simulink model "chapter2_4_1"  (R2022a)
settings: Solver=FixedStepAuto  StartTime=0.0  StopTime=8  FixedStep=1e-3  RelTol=1e-3
model workspace (MAT data in the model file):
  maxRandom = 1e-06
  minRandom = -1e-06
values from neighbouring files (symbols this model uses):
  Cb = 11e3    (= 11000)    [parameterLoadForchapter2_4.m]    (also in parameterLoadForchapter2_5.m)
  Cv = 5000    [parameterLoadForchapter2_4.m]    (also in parameterLoadForchapter2_5.m)
  d = 2.6    [parameterLoadForchapter2_4.m]    (also in parameterLoadForchapter2_5.m; parameter_load3.m)
  Jb = 927.8    [parameterLoadForchapter2_4.m]    (also in parameterLoadForchapter2_5.m)
  Jv = 3044    [parameterLoadForchapter2_4.m]    (also in parameterLoadForchapter2_5.m)
  Kb = 0.267e6    (= 267000)    [parameterLoadForchapter2_4.m]    (also in parameterLoadForchapter2_5.m)
  Kv = 1.5e6    (= 1500000)    [parameterLoadForchapter2_4.m]    (also in parameterLoadForchapter2_5.m)
  L = 210/2    (= 105)    [Figure2_18_and2_19.m]    (also in Figure2_20_and2_21.m; parameterLoadForchapter2_4.m = 15.6; parameterLoadForchapter2_5.m = 210; parameter_load3.m = 210)
  Ln = Lns(i)    [Figure2_14and2_15.m]    (also in Figure2_16and2_17.m; Mchapter2_4.m = LNs(i); Mchapter2_5.m = LN_set(i); parameterLoadForchapter2_5.m = 0.02)
  Ln1 = Ln    [Figure2_14and2_15.m]    (also in Figure2_16and2_17.m)
  Mb = 23000    [parameterLoadForchapter2_4.m]    (also in parameterLoadForchapter2_5.m)
  Mv = 4060    [parameterLoadForchapter2_4.m]    (also in parameterLoadForchapter2_5.m)
  mw = 1670    [parameterLoadForchapter2_4.m]    (also in parameterLoadForchapter2_5.m)
  Mw = 1670    [parameterLoadForchapter2_4.m]    (also in parameterLoadForchapter2_5.m)
  R = 400    [Figure2_3.m]    (also in parameterLoadForchapter2_4.m = 0.42; parameterLoadForchapter2_5.m = 0.42)
  r = 0.42    [parameterLoadForchapter2_4.m]    (also in parameterLoadForchapter2_5.m; parameter_load3.m)
  vkmh = 50    [parameterLoadForchapter2_4.m]    (also in parameterLoadForchapter2_5.m = 100)
settings Model: Creator=Spicydel  LastModifiedBy=Spicydel

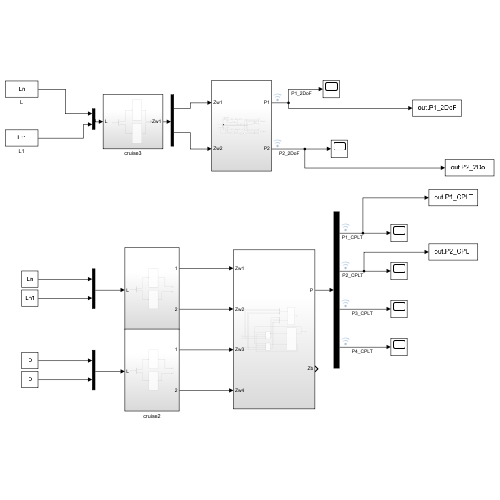
[thumbnail: Simulink's stored preview of the top-level diagram]
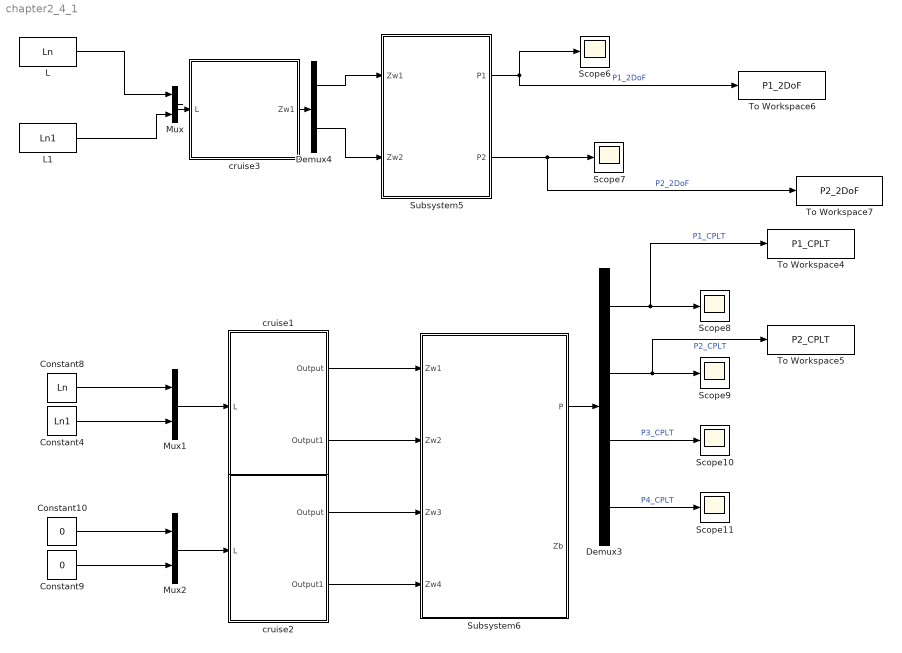
== system chapter2_4_1 ==
  Constant10 : Constant  Value=0
  Constant4 : Constant  Value=Ln1
  Constant8 : Constant  Value=Ln
  Constant9 : Constant  Value=0
  Demux3 : Demux
  Demux4 : Demux  Outputs=2
  L : Constant  Value=Ln
  L1 : Constant  Value=Ln1
  Mux : Mux  Inputs=2
  Mux1 : Mux  Inputs=2
  Mux2 : Mux  Inputs=2
  Scope{6..11} (6 alike) : Scope
  Subsystem5 : Subsystem
  Subsystem6 : Subsystem
  To Workspace4 : ToWorkspace  VariableName=P1_CPLT  SaveFormat=Timeseries  SampleTime=-1
  To Workspace5 : ToWorkspace  VariableName=P2_CPLT  SaveFormat=Timeseries  SampleTime=-1
  To Workspace6 : ToWorkspace  VariableName=P1_2DoF  SaveFormat=Timeseries  SampleTime=-1
  To Workspace7 : ToWorkspace  VariableName=P2_2DoF  SaveFormat=Timeseries  SampleTime=-1
  cruise1 : Subsystem
  cruise2 : Subsystem
  cruise3 : Subsystem
  wires:
  L/1 -> Mux/1
  Subsystem5/2(P2) -> To Workspace7/1, Scope7/1  "P2_2DoF"
  Subsystem5/1(P1) -> To Workspace6/1, Scope6/1  "P1_2DoF"
  Mux/1 -> cruise3/1(L)
  L1/1 -> Mux/2
  Demux4/1 -> Subsystem5/1(Zw1)
  Demux4/2 -> Subsystem5/2(Zw2)
  cruise1/1(Output) -> Subsystem6/1(Zw1)
  cruise1/2(Output1) -> Subsystem6/2(Zw2)
  cruise2/1(Output) -> Subsystem6/3(Zw3)
  cruise2/2(Output1) -> Subsystem6/4(Zw4)
  Constant4/1 -> Mux1/2
  Mux1/1 -> cruise1/1(L)
  Constant8/1 -> Mux1/1
  Constant10/1 -> Mux2/1
  Mux2/1 -> cruise2/1(L)
  Constant9/1 -> Mux2/2
  Demux3/4 -> Scope11/1  "P4_CPLT"
  Demux3/3 -> Scope10/1  "P3_CPLT"
  Demux3/2 -> To Workspace5/1, Scope9/1  "P2_CPLT"
  Demux3/1 -> To Workspace4/1, Scope8/1  "P1_CPLT"
  Subsystem6/1(P) -> Demux3/1
  cruise3/1(Zw1) -> Demux4/1

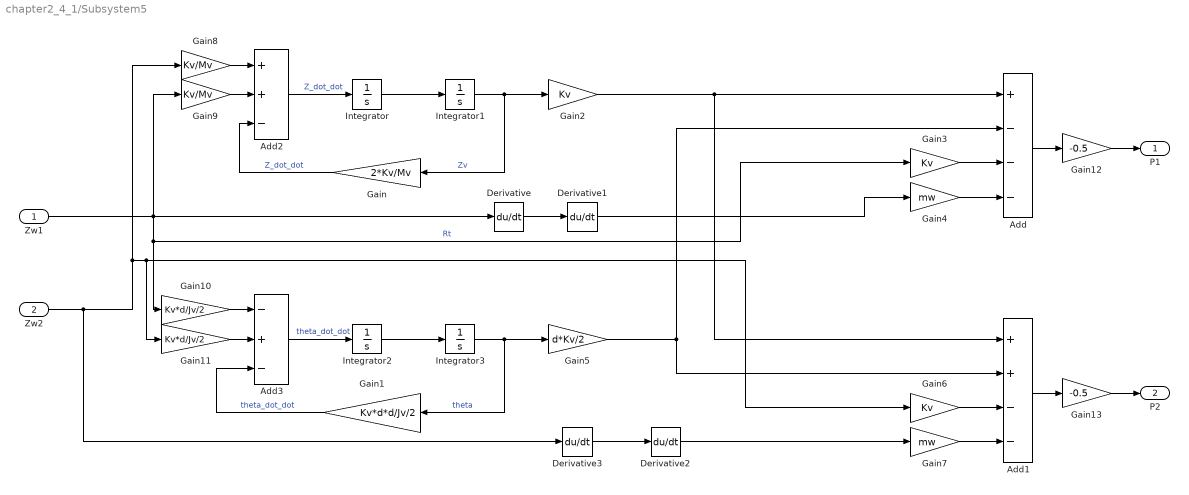
== system chapter2_4_1/Subsystem5 ==
  Zw1 : Inport
  Zw2 : Inport  Port=2
  Add : Sum  Inputs=+---
  Add1 : Sum  Inputs=++--
  Add2 : Sum  Inputs=++-
  Add3 : Sum  Inputs=-+-
  Derivative{,1..3} (4 alike) : Derivative
  Gain : Gain  Gain=2*Kv/Mv
  Gain1 : Gain  Gain=Kv*d*d/Jv/2
  Gain10 : Gain  Gain=Kv*d/Jv/2
  Gain11 : Gain  Gain=Kv*d/Jv/2
  Gain12 : Gain  Gain=-0.5
  Gain13 : Gain  Gain=-0.5
  Gain2 : Gain  Gain=Kv
  Gain3 : Gain  Gain=Kv
  Gain4 : Gain  Gain=mw
  Gain5 : Gain  Gain=d*Kv/2
  Gain6 : Gain  Gain=Kv
  Gain7 : Gain  Gain=mw
  Gain8 : Gain  Gain=Kv/Mv
  Gain9 : Gain  Gain=Kv/Mv
  Integrator{,1..3} (4 alike) : Integrator
  P1 : Outport
  P2 : Outport  Port=2
  wires:
  Gain13/1 -> P2/1
  Gain12/1 -> P1/1
  Gain11/1 -> Add3/2
  Gain10/1 -> Add3/1
  Gain1/1 -> Add3/3  "theta_dot_dot"
  Gain9/1 -> Add2/2
  Gain8/1 -> Add2/1
  Gain/1 -> Add2/3  "Z_dot_dot"
  Gain7/1 -> Add1/4
  Zw2/1 -> Derivative3/1, Gain8/1, Gain6/1, Gain11/1
  Gain6/1 -> Add1/3
  Gain4/1 -> Add/4
  Gain3/1 -> Add/3
  Zw1/1 -> Derivative/1, Gain3/1, Gain10/1, Gain9/1  "Rt"
  Add1/1 -> Gain13/1
  Add/1 -> Gain12/1
  Gain5/1 -> Add1/2, Add/2
  Gain2/1 -> Add/1, Add1/1
  Add3/1 -> Integrator2/1  "theta_dot_dot"
  Integrator3/1 -> Gain1/1, Gain5/1  "theta"
  Integrator2/1 -> Integrator3/1
  Add2/1 -> Integrator/1  "Z_dot_dot"
  Integrator1/1 -> Gain/1, Gain2/1  "Zv"
  Integrator/1 -> Integrator1/1
  Derivative/1 -> Derivative1/1
  Derivative1/1 -> Gain4/1
  Derivative2/1 -> Gain7/1
  Derivative3/1 -> Derivative2/1

== system chapter2_4_1/Subsystem6 ==
  Zw1 : Inport
  Zw2 : Inport  Port=2
  Zw3 : Inport  Port=3
  Zw4 : Inport  Port=4
  FrontTrans : Subsystem
  Mux : Mux
  Mux1 : Mux
  RearTrans : Subsystem
  Subsystem : Subsystem
  Subsystem2 : Subsystem
  P : Outport
  Zb : Outport  Port=2
  wires:
  Subsystem/1(P) -> P/1
  Mux1/1 -> Subsystem/2(Z&theta)
  Mux/1 -> Subsystem/1(Zw)
  RearTrans/2(theta_v2) -> Mux1/4
  FrontTrans/2(theta_v1) -> Mux1/2
  Zw2/1 -> FrontTrans/4(Zw2), Mux/2
  Zw1/1 -> FrontTrans/3(Zw1), Mux/1
  Zw3/1 -> RearTrans/3(Zw3), Mux/3
  Subsystem2/2(theta_b) -> RearTrans/2(theta_b), FrontTrans/2(theta_b)
  Zw4/1 -> RearTrans/4(Zw4), Mux/4
  Subsystem2/1(Zb) -> FrontTrans/1(Zb), RearTrans/1(Zb), Zb/1  "Zb"
  FrontTrans/1(Zv1) -> Subsystem2/1(Zv1), Mux1/1
  RearTrans/1(Zv2) -> Subsystem2/2(Zv2), Mux1/3

== system chapter2_4_1/cruise1 ==
  L : Inport
  Demux : Demux  Outputs=2
  Subsystem1 : Subsystem
  Subsystem2 : Subsystem
  Output : Outport
  Output1 : Outport  Port=2
  wires:
  Subsystem2/1(Output) -> Output1/1
  Subsystem1/1(Output) -> Output/1
  Demux/2 -> Subsystem2/1(In1)
  Demux/1 -> Subsystem1/1(In1)
  L/1 -> Demux/1

== system chapter2_4_1/cruise2 ==
  L : Inport
  Demux : Demux  Outputs=2
  Subsystem1 : Subsystem
  Subsystem2 : Subsystem
  Output : Outport
  Output1 : Outport  Port=2
  wires:
  L/1 -> Demux/1
  Demux/1 -> Subsystem1/1(In1)
  Demux/2 -> Subsystem2/1(In1)
  Subsystem1/1(Output) -> Output/1
  Subsystem2/1(Output) -> Output1/1

== system chapter2_4_1/cruise3 ==
  L : Inport
  Demux : Demux  Outputs=2
  Mux : Mux  Inputs=2
  Subsystem1 : Subsystem
  Subsystem2 : Subsystem
  Zw1 : Outport
  wires:
  L/1 -> Demux/1
  Demux/1 -> Subsystem1/1(In1)
  Demux/2 -> Subsystem2/1(In1)
  Subsystem1/1(Output) -> Mux/1
  Subsystem2/1(Output) -> Mux/2
  Mux/1 -> Zw1/1

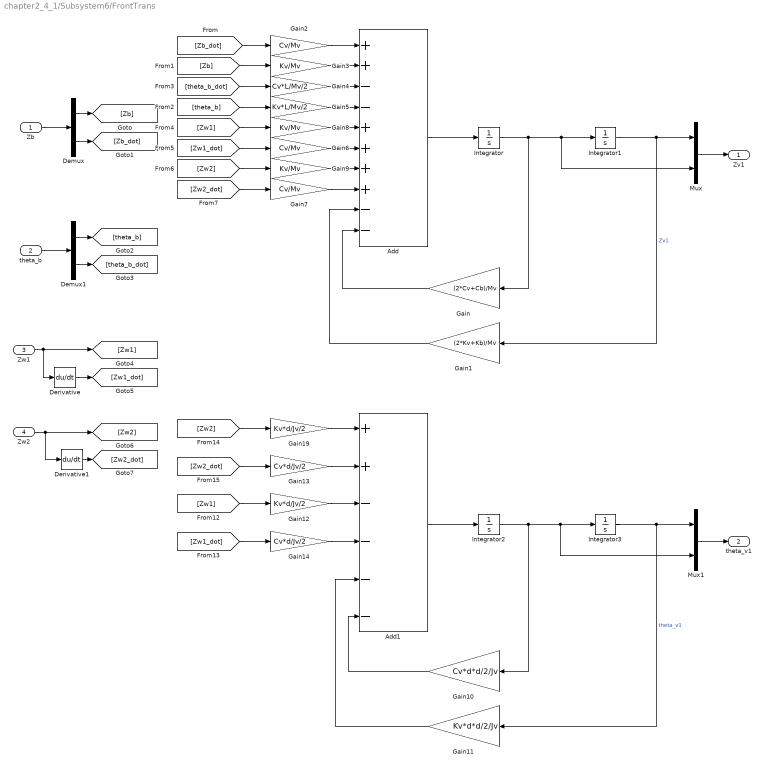
== system chapter2_4_1/Subsystem6/FrontTrans ==
  Zb : Inport
  theta_b : Inport  Port=2
  Zw1 : Inport  Port=3
  Zw2 : Inport  Port=4
  Add : Sum  Inputs=++--++++--
  Add1 : Sum  Inputs=++----
  Demux : Demux  Outputs=2
  Demux1 : Demux  Outputs=2
  Derivative : Derivative
  Derivative1 : Derivative
  Gain : Gain  Gain=(2*Cv+Cb)/Mv
  Gain1 : Gain  Gain=(2*Kv+Kb)/Mv
  Gain10 : Gain  Gain=Cv*d*d/2/Jv
  Gain11 : Gain  Gain=Kv*d*d/2/Jv
  Gain12 : Gain  Gain=Kv*d/Jv/2
  Gain13 : Gain  Gain=Cv*d/Jv/2
  Gain14 : Gain  Gain=Cv*d/Jv/2
  Gain19 : Gain  Gain=Kv*d/Jv/2
  Gain2 : Gain  Gain=Cv/Mv
  Gain3 : Gain  Gain=Kv/Mv
  Gain4 : Gain  Gain=Cv*L/Mv/2
  Gain5 : Gain  Gain=Kv*L/Mv/2
  Gain6 : Gain  Gain=Cv/Mv
  Gain7 : Gain  Gain=Cv/Mv
  Gain8 : Gain  Gain=Kv/Mv
  Gain9 : Gain  Gain=Kv/Mv
  Integrator{,1..3} (4 alike) : Integrator
  Mux : Mux  Inputs=2
  Mux1 : Mux  Inputs=2
  Zv1 : Outport
  theta_v1 : Outport  Port=2
  wires:
  Derivative1/1 -> [Zw2_dot]
  Zw2/1 -> Derivative1/1, [Zw2]
  Derivative/1 -> [Zw1_dot]
  Integrator2/1 -> Gain10/1, Integrator3/1, Mux1/2
  Integrator3/1 -> Gain11/1, Mux1/1  "theta_v1"
  Mux1/1 -> theta_v1/1
  Gain14/1 -> Add1/4
  Gain13/1 -> Add1/2
  Gain12/1 -> Add1/3
  Gain19/1 -> Add1/1
  Add1/1 -> Integrator2/1
  Gain10/1 -> Add1/6
  Gain11/1 -> Add1/5
  [Zw2] -> Gain19/1
  [Zw2_dot] -> Gain13/1
  [Zw1_dot] -> Gain14/1
  [Zw1] -> Gain12/1
  Gain7/1 -> Add/8
  Gain9/1 -> Add/7
  Gain6/1 -> Add/6
  Gain8/1 -> Add/5
  [Zw1] -> Gain8/1
  [Zw1_dot] -> Gain6/1
  [Zw2_dot] -> Gain7/1
  [Zw2] -> Gain9/1
  Gain5/1 -> Add/4
  [theta_b] -> Gain5/1
  Gain4/1 -> Add/3
  [theta_b_dot] -> Gain4/1
  Gain3/1 -> Add/2
  [Zb] -> Gain3/1
  Gain2/1 -> Add/1
  [Zb_dot] -> Gain2/1
  Gain1/1 -> Add/9
  Gain/1 -> Add/10
  Zw1/1 -> Derivative/1, [Zw1]
  Mux/1 -> Zv1/1
  Integrator1/1 -> Mux/1, Gain1/1  "Zv1"
  Add/1 -> Integrator/1
  Integrator/1 -> Integrator1/1, Mux/2, Gain/1
  Demux1/2 -> [theta_b_dot]
  Demux1/1 -> [theta_b]
  Demux/2 -> [Zb_dot]
  Demux/1 -> [Zb]
  theta_b/1 -> Demux1/1
  Zb/1 -> Demux/1

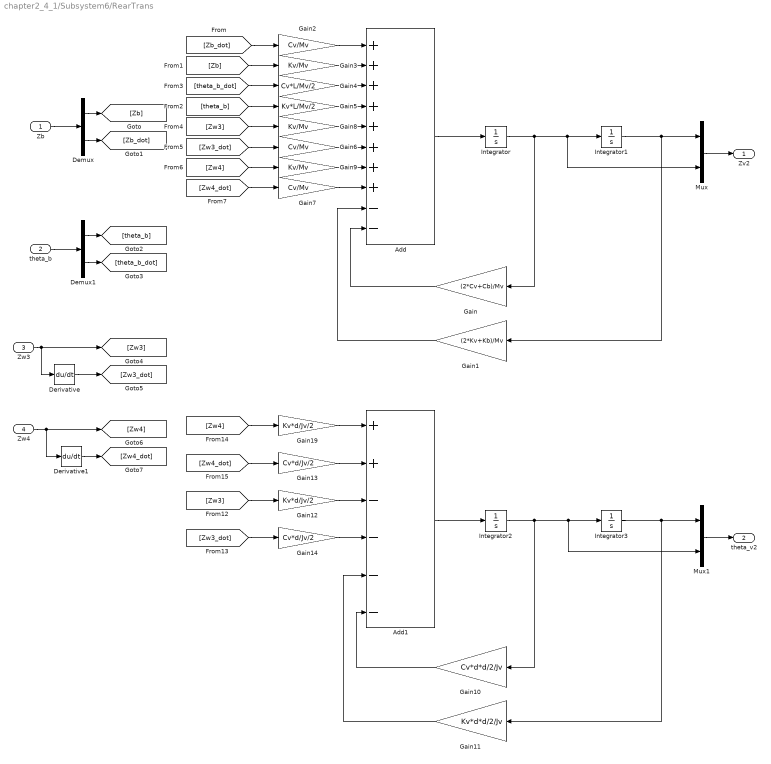
== system chapter2_4_1/Subsystem6/RearTrans ==
  Zb : Inport
  theta_b : Inport  Port=2
  Zw3 : Inport  Port=3
  Zw4 : Inport  Port=4
  Add : Sum  Inputs=++++++++--
  Add1 : Sum  Inputs=++----
  Demux : Demux  Outputs=2
  Demux1 : Demux  Outputs=2
  Derivative : Derivative
  Derivative1 : Derivative
  Gain : Gain  Gain=(2*Cv+Cb)/Mv
  Gain1 : Gain  Gain=(2*Kv+Kb)/Mv
  Gain10 : Gain  Gain=Cv*d*d/2/Jv
  Gain11 : Gain  Gain=Kv*d*d/2/Jv
  Gain12 : Gain  Gain=Kv*d/Jv/2
  Gain13 : Gain  Gain=Cv*d/Jv/2
  Gain14 : Gain  Gain=Cv*d/Jv/2
  Gain19 : Gain  Gain=Kv*d/Jv/2
  Gain2 : Gain  Gain=Cv/Mv
  Gain3 : Gain  Gain=Kv/Mv
  Gain4 : Gain  Gain=Cv*L/Mv/2
  Gain5 : Gain  Gain=Kv*L/Mv/2
  Gain6 : Gain  Gain=Cv/Mv
  Gain7 : Gain  Gain=Cv/Mv
  Gain8 : Gain  Gain=Kv/Mv
  Gain9 : Gain  Gain=Kv/Mv
  Integrator{,1..3} (4 alike) : Integrator
  Mux : Mux  Inputs=2
  Mux1 : Mux  Inputs=2
  Zv2 : Outport
  theta_v2 : Outport  Port=2
  wires:
  Derivative/1 -> [Zw3_dot]
  Mux1/1 -> theta_v2/1
  Integrator3/1 -> Gain11/1, Mux1/1
  Integrator2/1 -> Integrator3/1, Mux1/2, Gain10/1
  Zb/1 -> Demux/1
  theta_b/1 -> Demux1/1
  Demux/1 -> [Zb]
  Demux/2 -> [Zb_dot]
  Demux1/1 -> [theta_b]
  Demux1/2 -> [theta_b_dot]
  Integrator/1 -> Gain/1, Mux/2, Integrator1/1
  Add/1 -> Integrator/1
  Integrator1/1 -> Gain1/1, Mux/1
  Mux/1 -> Zv2/1
  Zw3/1 -> [Zw3], Derivative/1
  Derivative1/1 -> [Zw4_dot]
  Zw4/1 -> [Zw4], Derivative1/1
  Gain/1 -> Add/10
  Gain1/1 -> Add/9
  [Zb_dot] -> Gain2/1
  Gain2/1 -> Add/1
  [Zb] -> Gain3/1
  Gain3/1 -> Add/2
  [theta_b_dot] -> Gain4/1
  Gain4/1 -> Add/3
  [theta_b] -> Gain5/1
  Gain5/1 -> Add/4
  [Zw4] -> Gain9/1
  [Zw4_dot] -> Gain7/1
  [Zw3_dot] -> Gain6/1
  [Zw3] -> Gain8/1
  Gain8/1 -> Add/5
  Gain6/1 -> Add/6
  Gain9/1 -> Add/7
  Gain7/1 -> Add/8
  [Zw3] -> Gain12/1
  [Zw3_dot] -> Gain14/1
  [Zw4_dot] -> Gain13/1
  [Zw4] -> Gain19/1
  Gain11/1 -> Add1/5
  Gain10/1 -> Add1/6
  Add1/1 -> Integrator2/1
  Gain19/1 -> Add1/1
  Gain12/1 -> Add1/3
  Gain13/1 -> Add1/2
  Gain14/1 -> Add1/4

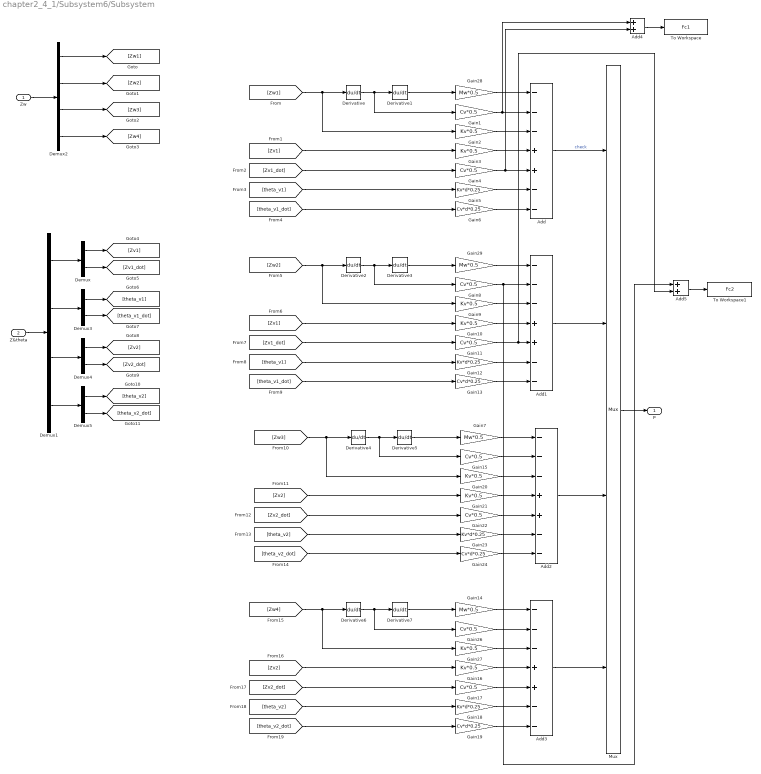
== system chapter2_4_1/Subsystem6/Subsystem ==
  Zw : Inport
  Z&theta : Inport  Port=2
  Add{,1..3} (4 alike) : Sum  Inputs=---++--
  Add4 : Sum
  Add5 : Sum
  Demux{,3..5} (4 alike) : Demux  Outputs=2
  Demux1 : Demux
  Demux2 : Demux
  Derivative{,1..7} (8 alike) : Derivative
  Gain{1,4,8,11,15,17,22,26} (8 alike) : Gain  Gain=Cv*0.5
  Gain{2..3,9..10,16,20..21,27} (8 alike) : Gain  Gain=Kv*0.5
  Gain{5,12,18,23} (4 alike) : Gain  Gain=Kv*d*0.25
  Gain{6,13,19,24} (4 alike) : Gain  Gain=Cv*d*0.25
  Gain{7,14,28..29} (4 alike) : Gain  Gain=Mw*0.5
  Mux : Mux
  To Workspace : ToWorkspace  VariableName=Fc1  SaveFormat=Timeseries  SampleTime=-1
  To Workspace1 : ToWorkspace  VariableName=Fc2  SaveFormat=Timeseries  SampleTime=-1
  P : Outport
  wires:
  Add5/1 -> To Workspace1/1
  Add4/1 -> To Workspace/1
  Mux/1 -> P/1
  [Zw3] -> Derivative4/1, Gain20/1
  Derivative4/1 -> Gain15/1, Derivative5/1
  Derivative5/1 -> Gain7/1
  Gain7/1 -> Add2/1
  Gain15/1 -> Add2/2
  Gain20/1 -> Add2/3
  Gain21/1 -> Add2/4
  [Zv2] -> Gain21/1
  Gain22/1 -> Add2/5
  [Zv2_dot] -> Gain22/1
  Gain23/1 -> Add2/6
  Gain24/1 -> Add2/7
  [theta_v2] -> Gain23/1
  [theta_v2_dot] -> Gain24/1
  Add2/1 -> Mux/3
  Add3/1 -> Mux/4
  [theta_v2_dot] -> Gain19/1
  [theta_v2] -> Gain18/1
  Gain19/1 -> Add3/7
  Gain18/1 -> Add3/6
  [Zv2_dot] -> Gain17/1
  Gain17/1 -> Add3/5
  [Zv2] -> Gain16/1
  Gain16/1 -> Add3/4
  Gain27/1 -> Add3/3
  Gain26/1 -> Add3/2
  Gain14/1 -> Add3/1
  Derivative7/1 -> Gain14/1
  Derivative6/1 -> Derivative7/1, Gain26/1
  [Zw4] -> Derivative6/1, Gain27/1
  [Zw2] -> Derivative2/1, Gain9/1
  Derivative2/1 -> Gain8/1, Derivative3/1
  Derivative3/1 -> Gain29/1
  Gain29/1 -> Add1/1
  Gain8/1 -> Add1/2, Add5/1
  Gain9/1 -> Add1/3
  Gain10/1 -> Add1/4
  [Zv1] -> Gain10/1
  Gain11/1 -> Add1/5, Add5/2
  [Zv1_dot] -> Gain11/1
  Gain12/1 -> Add1/6
  Gain13/1 -> Add1/7
  [theta_v1] -> Gain12/1
  [theta_v1_dot] -> Gain13/1
  Add1/1 -> Mux/2
  Add/1 -> Mux/1  "check"
  [theta_v1_dot] -> Gain6/1
  [theta_v1] -> Gain5/1
  Gain6/1 -> Add/7
  Gain5/1 -> Add/6
  [Zv1_dot] -> Gain4/1
  Gain4/1 -> Add/5, Add4/2
  [Zv1] -> Gain3/1
  Gain3/1 -> Add/4
  Gain2/1 -> Add/3
  Gain1/1 -> Add/2, Add4/1
  Gain28/1 -> Add/1
  Derivative1/1 -> Gain28/1
  Derivative/1 -> Derivative1/1, Gain1/1
  [Zw1] -> Derivative/1, Gain2/1
  Demux5/1 -> [theta_v2]
  Demux5/2 -> [theta_v2_dot]
  Demux4/1 -> [Zv2]
  Demux4/2 -> [Zv2_dot]
  Demux3/2 -> [theta_v1_dot]
  Demux3/1 -> [theta_v1]
  Demux/2 -> [Zv1_dot]
  Demux/1 -> [Zv1]
  Demux1/4 -> Demux5/1
  Demux1/3 -> Demux4/1
  Demux1/2 -> Demux3/1
  Demux1/1 -> Demux/1
  Demux2/4 -> [Zw4]
  Demux2/3 -> [Zw3]
  Demux2/2 -> [Zw2]
  Demux2/1 -> [Zw1]
  Z&theta/1 -> Demux1/1
  Zw/1 -> Demux2/1

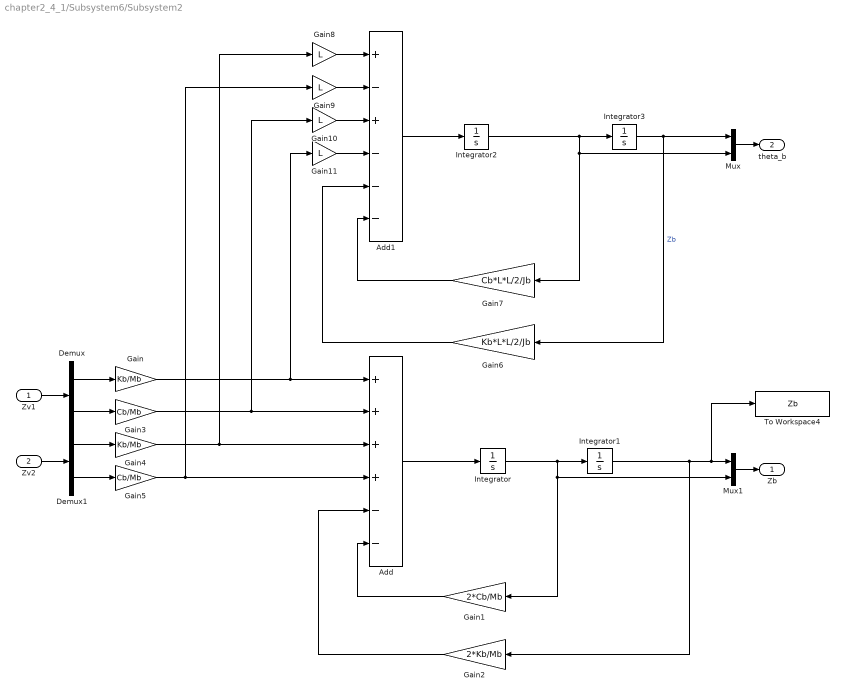
== system chapter2_4_1/Subsystem6/Subsystem2 ==
  Zv1 : Inport
  Zv2 : Inport  Port=2
  Add : Sum  Inputs=++++--
  Add1 : Sum  Inputs=+-+---
  Demux : Demux  Outputs=2
  Demux1 : Demux  Outputs=2
  Gain : Gain  Gain=Kb/Mb
  Gain1 : Gain  Gain=2*Cb/Mb
  Gain{8..11} (4 alike) : Gain  Gain=L
  Gain2 : Gain  Gain=2*Kb/Mb
  Gain3 : Gain  Gain=Cb/Mb
  Gain4 : Gain  Gain=Kb/Mb
  Gain5 : Gain  Gain=Cb/Mb
  Gain6 : Gain  Gain=Kb*L*L/2/Jb
  Gain7 : Gain  Gain=Cb*L*L/2/Jb
  Integrator{,1..3} (4 alike) : Integrator
  Mux : Mux  Inputs=2
  Mux1 : Mux  Inputs=2
  To Workspace4 : ToWorkspace  VariableName=Zb  SaveFormat=Timeseries  SampleTime=-1
  Zb : Outport
  theta_b : Outport  Port=2
  wires:
  Demux1/2 -> Gain5/1
  Demux1/1 -> Gain4/1
  Zv2/1 -> Demux1/1
  Demux/2 -> Gain3/1
  Demux/1 -> Gain/1
  Zv1/1 -> Demux/1
  Mux1/1 -> Zb/1
  Mux/1 -> theta_b/1
  Gain11/1 -> Add1/4
  Gain10/1 -> Add1/3
  Gain9/1 -> Add1/2
  Gain8/1 -> Add1/1
  Gain3/1 -> Add/2, Gain10/1
  Gain6/1 -> Add1/5
  Gain7/1 -> Add1/6
  Add1/1 -> Integrator2/1
  Integrator3/1 -> Gain6/1, Mux/1  "Zb"
  Integrator2/1 -> Integrator3/1, Gain7/1, Mux/2
  Gain5/1 -> Add/4, Gain9/1
  Gain4/1 -> Add/3, Gain8/1
  Gain/1 -> Add/1, Gain11/1
  Integrator1/1 -> Gain2/1, Mux1/1, To Workspace4/1
  Integrator/1 -> Integrator1/1, Gain1/1, Mux1/2
  Gain2/1 -> Add/5
  Add/1 -> Integrator/1
  Gain1/1 -> Add/6

== system chapter2_4_1/cruise1/Subsystem1 ==
  In1 : Inport
  Constant : Constant  Value=0
  Gain8 : Gain  Gain=2/pi
  Subsystem : Subsystem
  Switch : Switch  Criteria=u2 ~= 0  SaturateOnIntegerOverflow=off  InputSameDT=off
  Output : Outport
  wires:
  Constant/1 -> Switch/3
  In1/1 -> Gain8/1, Switch/2, Subsystem/1(L)
  Gain8/1 -> Subsystem/2(L0)
  Switch/1 -> Output/1
  Subsystem/1(Output) -> Switch/1

== system chapter2_4_1/cruise1/Subsystem2 ==
  In1 : Inport
  Constant : Constant  Value=0
  Gain8 : Gain  Gain=2/pi
  Subsystem : Subsystem
  Switch : Switch  Criteria=u2 ~= 0  SaturateOnIntegerOverflow=off  InputSameDT=off
  Output : Outport
  wires:
  Gain8/1 -> Subsystem/2(L0)
  In1/1 -> Subsystem/1(L), Switch/2, Gain8/1
  Subsystem/1(Output) -> Switch/1
  Constant/1 -> Switch/3
  Switch/1 -> Output/1

== system chapter2_4_1/cruise2/Subsystem1 ==
  In1 : Inport
  Constant : Constant  Value=0
  Demux : Demux  Outputs=2
  Gain8 : Gain  Gain=2/pi
  Mux : Mux  Inputs=2
  Mux1 : Mux  Inputs=2
  Subsystem : Subsystem
  Switch : Switch  Criteria=u2 ~= 0  SaturateOnIntegerOverflow=off  InputSameDT=off
  Terminator : Terminator
  Output : Outport
  wires:
  Demux/2 -> Terminator/1
  Demux/1 -> Output/1
  Gain8/1 -> Subsystem/2(L0)
  In1/1 -> Subsystem/1(L), Switch/2, Gain8/1
  Switch/1 -> Demux/1
  Subsystem/1(Output) -> Mux/1
  Constant/1 -> Mux1/2, Mux1/1
  Subsystem/2(Rt_curise_dot_dot) -> Mux/2
  Mux/1 -> Switch/1
  Mux1/1 -> Switch/3

== system chapter2_4_1/cruise2/Subsystem2 ==
  In1 : Inport
  Constant : Constant  Value=0
  Demux : Demux  Outputs=2
  Gain8 : Gain  Gain=2/pi
  Mux : Mux  Inputs=2
  Mux1 : Mux  Inputs=2
  Subsystem : Subsystem
  Switch : Switch  Criteria=u2 ~= 0  SaturateOnIntegerOverflow=off  InputSameDT=off
  Terminator : Terminator
  Output : Outport
  wires:
  Demux/2 -> Terminator/1
  Demux/1 -> Output/1
  Mux1/1 -> Switch/3
  Mux/1 -> Switch/1
  Subsystem/2(Rt_curise_dot_dot) -> Mux/2
  Constant/1 -> Mux1/1, Mux1/2
  Subsystem/1(Output) -> Mux/1
  Switch/1 -> Demux/1
  In1/1 -> Gain8/1, Switch/2, Subsystem/1(L)
  Gain8/1 -> Subsystem/2(L0)

== system chapter2_4_1/cruise3/Subsystem1 ==
  In1 : Inport
  Constant : Constant  Value=0
  Gain8 : Gain  Gain=2/pi
  Subsystem : Subsystem
  Switch : Switch  Criteria=u2 ~= 0  SaturateOnIntegerOverflow=off  InputSameDT=off
  Output : Outport
  wires:
  Gain8/1 -> Subsystem/2(L0)
  In1/1 -> Subsystem/1(L), Switch/2, Gain8/1
  Switch/1 -> Output/1
  Constant/1 -> Switch/3
  Subsystem/1(Output) -> Switch/1

== system chapter2_4_1/cruise3/Subsystem2 ==
  In1 : Inport
  Constant : Constant  Value=0
  Gain8 : Gain  Gain=2/pi
  Subsystem : Subsystem
  Switch : Switch  Criteria=u2 ~= 0  SaturateOnIntegerOverflow=off  InputSameDT=off
  Output : Outport
  wires:
  Constant/1 -> Switch/3
  Subsystem/1(Output) -> Switch/1
  Switch/1 -> Output/1
  In1/1 -> Gain8/1, Switch/2, Subsystem/1(L)
  Gain8/1 -> Subsystem/2(L0)

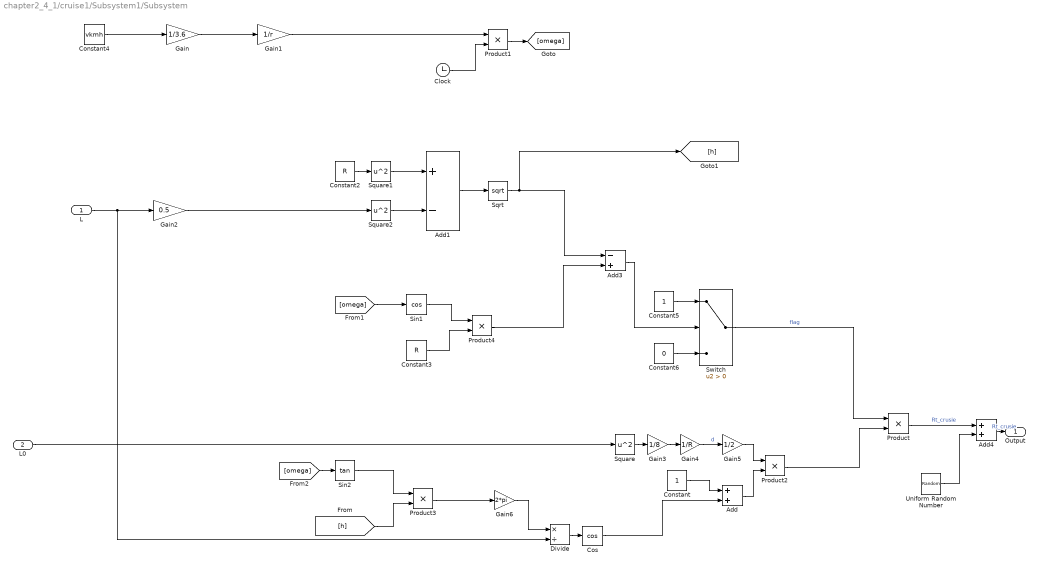
== system chapter2_4_1/cruise1/Subsystem1/Subsystem ==
  L : Inport
  L0 : Inport  Port=2
  Add : Sum
  Add1 : Sum  Inputs=+-
  Add3 : Sum  Inputs=-+
  Add4 : Sum
  Clock : Clock
  Constant : Constant
  Constant2 : Constant  Value=R
  Constant3 : Constant  Value=R
  Constant4 : Constant  Value=vkmh
  Constant5 : Constant
  Constant6 : Constant  Value=0
  Cos : Trigonometry  Operator=cos
  Divide : Product  Inputs=*/
  Gain : Gain  Gain=1/3.6
  Gain1 : Gain  Gain=1/r
  Gain2 : Gain  Gain=0.5
  Gain3 : Gain  Gain=1/8
  Gain4 : Gain  Gain=1/R
  Gain5 : Gain  Gain=1/2
  Gain6 : Gain  Gain=2*pi
  Product{,1..4} (5 alike) : Product
  Sin1 : Trigonometry  Operator=cos
  Sin2 : Trigonometry  Operator=tan
  Sqrt : Sqrt
  Square : Math  Operator=square
  Square1 : Math  Operator=square
  Square2 : Math  Operator=square
  Switch : Switch  Criteria=u2 > Threshold  SaturateOnIntegerOverflow=off  InputSameDT=off
  Uniform Random Number : UniformRandomNumber  Minimum=minRandom  Maximum=maxRandom  SampleTime=1e-3
  Output : Outport
  wires:
  L/1 -> Gain2/1, Divide/2
  Constant4/1 -> Gain/1
  Gain6/1 -> Divide/1
  [omega] -> Sin2/1
  Gain2/1 -> Square2/1
  L0/1 -> Square/1
  Constant/1 -> Add/1
  Cos/1 -> Add/2
  Gain5/1 -> Product2/1
  Sin2/1 -> Product3/1
  Product3/1 -> Gain6/1
  Gain1/1 -> Product1/1
  Product2/1 -> Product/2
  Sqrt/1 -> Add3/1, [h]
  Product/1 -> Add4/1  "Rt_crusie"
  Add/1 -> Product2/2
  Sin1/1 -> Product4/1
  Square1/1 -> Add1/1
  Switch/1 -> Product/1  "flag"
  Square2/1 -> Add1/2
  Constant5/1 -> Switch/1
  Gain4/1 -> Gain5/1  "d"
  Add3/1 -> Switch/2
  Constant3/1 -> Product4/2
  [omega] -> Sin1/1
  [h] -> Product3/2
  Constant6/1 -> Switch/3
  Square/1 -> Gain3/1
  Constant2/1 -> Square1/1
  Product4/1 -> Add3/2
  Gain/1 -> Gain1/1
  Divide/1 -> Cos/1
  Gain3/1 -> Gain4/1
  Add1/1 -> Sqrt/1
  Product1/1 -> [omega]
  Clock/1 -> Product1/2
  Uniform Random Number/1 -> Add4/2
  Add4/1 -> Output/1  "Rt_crusie"

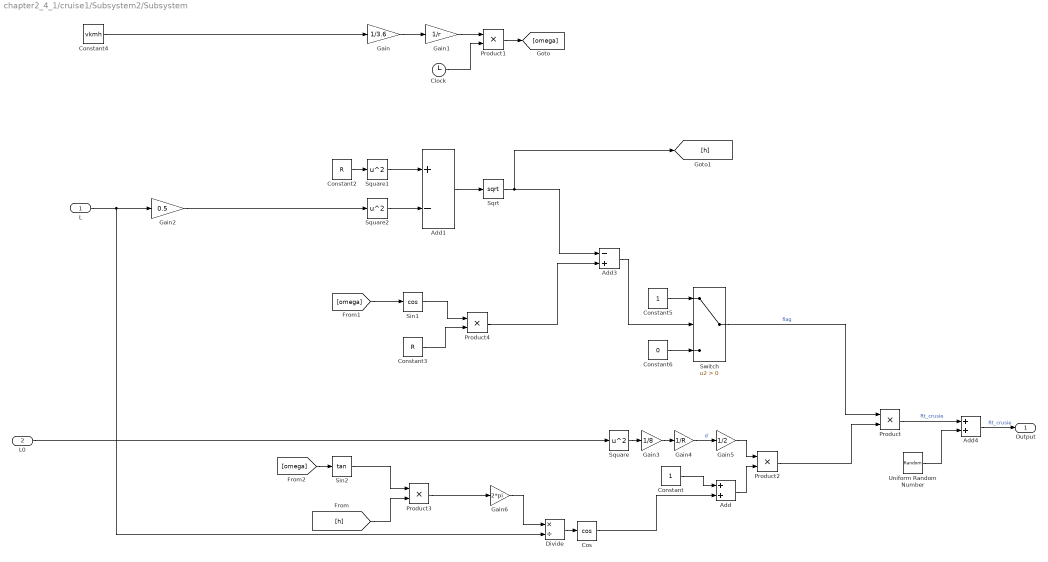
== system chapter2_4_1/cruise1/Subsystem2/Subsystem ==
  L : Inport
  L0 : Inport  Port=2
  Add : Sum
  Add1 : Sum  Inputs=+-
  Add3 : Sum  Inputs=-+
  Add4 : Sum
  Clock : Clock
  Constant : Constant
  Constant2 : Constant  Value=R
  Constant3 : Constant  Value=R
  Constant4 : Constant  Value=vkmh
  Constant5 : Constant
  Constant6 : Constant  Value=0
  Cos : Trigonometry  Operator=cos
  Divide : Product  Inputs=*/
  Gain : Gain  Gain=1/3.6
  Gain1 : Gain  Gain=1/r
  Gain2 : Gain  Gain=0.5
  Gain3 : Gain  Gain=1/8
  Gain4 : Gain  Gain=1/R
  Gain5 : Gain  Gain=1/2
  Gain6 : Gain  Gain=2*pi
  Product{,1..4} (5 alike) : Product
  Sin1 : Trigonometry  Operator=cos
  Sin2 : Trigonometry  Operator=tan
  Sqrt : Sqrt
  Square : Math  Operator=square
  Square1 : Math  Operator=square
  Square2 : Math  Operator=square
  Switch : Switch  Criteria=u2 > Threshold  SaturateOnIntegerOverflow=off  InputSameDT=off
  Uniform Random Number : UniformRandomNumber  Minimum=minRandom  Maximum=maxRandom  Seed=1  SampleTime=1e-3
  Output : Outport
  wires:
  Clock/1 -> Product1/2
  Product1/1 -> [omega]
  Add1/1 -> Sqrt/1
  Gain3/1 -> Gain4/1
  Divide/1 -> Cos/1
  Gain/1 -> Gain1/1
  Product4/1 -> Add3/2
  Constant2/1 -> Square1/1
  Square/1 -> Gain3/1
  Constant6/1 -> Switch/3
  [h] -> Product3/2
  [omega] -> Sin1/1
  Constant3/1 -> Product4/2
  Add3/1 -> Switch/2
  Gain4/1 -> Gain5/1  "d"
  Constant5/1 -> Switch/1
  Square2/1 -> Add1/2
  Switch/1 -> Product/1  "flag"
  Square1/1 -> Add1/1
  Sin1/1 -> Product4/1
  Add/1 -> Product2/2
  Product/1 -> Add4/1  "Rt_crusie"
  Sqrt/1 -> [h], Add3/1
  Product2/1 -> Product/2
  Gain1/1 -> Product1/1
  Product3/1 -> Gain6/1
  Sin2/1 -> Product3/1
  Gain5/1 -> Product2/1
  Cos/1 -> Add/2
  Constant/1 -> Add/1
  L0/1 -> Square/1
  Gain2/1 -> Square2/1
  [omega] -> Sin2/1
  Gain6/1 -> Divide/1
  Constant4/1 -> Gain/1
  L/1 -> Divide/2, Gain2/1
  Uniform Random Number/1 -> Add4/2
  Add4/1 -> Output/1  "Rt_crusie"

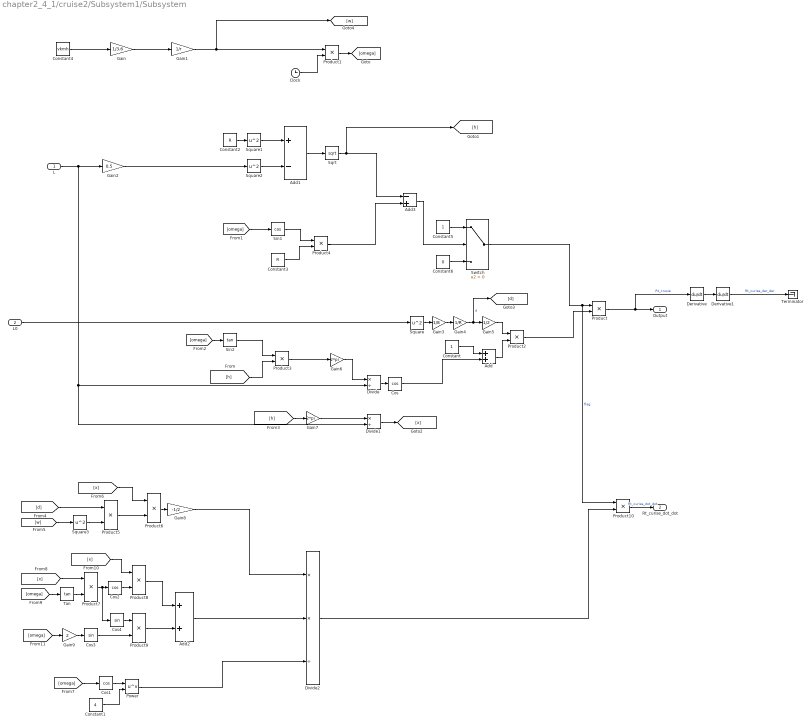
== system chapter2_4_1/cruise2/Subsystem1/Subsystem ==
  L : Inport
  L0 : Inport  Port=2
  Add : Sum
  Add1 : Sum  Inputs=+-
  Add2 : Sum
  Add3 : Sum  Inputs=-+
  Clock : Clock
  Constant : Constant
  Constant1 : Constant  Value=4
  Constant2 : Constant  Value=R
  Constant3 : Constant  Value=R
  Constant4 : Constant  Value=vkmh
  Constant5 : Constant
  Constant6 : Constant  Value=0
  Cos : Trigonometry  Operator=cos
  Cos1 : Trigonometry  Operator=cos
  Cos2 : Trigonometry  Operator=cos
  Cos3 : Trigonometry
  Cos4 : Trigonometry
  Derivative : Derivative
  Derivative1 : Derivative
  Divide : Product  Inputs=*/
  Divide1 : Product  Inputs=*/
  Divide2 : Product  Inputs=**/
  Gain : Gain  Gain=1/3.6
  Gain1 : Gain  Gain=1/r
  Gain2 : Gain  Gain=0.5
  Gain3 : Gain  Gain=1/8
  Gain4 : Gain  Gain=1/R
  Gain5 : Gain  Gain=1/2
  Gain6 : Gain  Gain=2*pi
  Gain7 : Gain  Gain=2*pi
  Gain8 : Gain  Gain=-1/2
  Gain9 : Gain  Gain=2
  Power : Math  Operator=pow
  Product{,1..10} (11 alike) : Product
  Sin1 : Trigonometry  Operator=cos
  Sin2 : Trigonometry  Operator=tan
  Sqrt : Sqrt
  Square{,1..3} (4 alike) : Math  Operator=square
  Switch : Switch  Criteria=u2 > Threshold  SaturateOnIntegerOverflow=off  InputSameDT=off
  Tan : Trigonometry  Operator=tan
  Terminator : Terminator
  Output : Outport
  Rt_curise_dot_dot : Outport  Port=2
  wires:
  Clock/1 -> Product1/2
  Product1/1 -> [omega]
  Add1/1 -> Sqrt/1
  Gain3/1 -> Gain4/1
  Divide/1 -> Cos/1
  Gain/1 -> Gain1/1
  Product4/1 -> Add3/2
  Constant2/1 -> Square1/1
  Square/1 -> Gain3/1
  Constant6/1 -> Switch/3
  [h] -> Product3/2
  [omega] -> Sin1/1
  Constant3/1 -> Product4/2
  Add3/1 -> Switch/2
  Gain4/1 -> [d], Gain5/1  "d"
  Constant5/1 -> Switch/1
  Square2/1 -> Add1/2
  Switch/1 -> Product10/1, Product/1  "flag"
  Square1/1 -> Add1/1
  Sin1/1 -> Product4/1
  Add/1 -> Product2/2
  Product/1 -> Derivative/1, Output/1  "Rt_crusie"
  Sqrt/1 -> [h], Add3/1
  Product2/1 -> Product/2
  Gain1/1 -> Product1/1, [w]
  Product3/1 -> Gain6/1
  Sin2/1 -> Product3/1
  Gain5/1 -> Product2/1
  Cos/1 -> Add/2
  Constant/1 -> Add/1
  L0/1 -> Square/1
  Gain2/1 -> Square2/1
  [omega] -> Sin2/1
  Gain6/1 -> Divide/1
  Constant4/1 -> Gain/1
  L/1 -> Divide/2, Divide1/2, Gain2/1
  [h] -> Gain7/1
  Gain7/1 -> Divide1/1
  Divide1/1 -> [x]
  [w] -> Square3/1
  Square3/1 -> Product5/2
  [d] -> Product5/1
  Product5/1 -> Product6/2
  [x] -> Product6/1
  Product6/1 -> Gain8/1
  [omega] -> Cos1/1
  Cos1/1 -> Power/1
  Constant1/1 -> Power/2
  Power/1 -> Divide2/3
  [omega] -> Tan/1
  Tan/1 -> Product7/2
  [x] -> Product7/1
  Product7/1 -> Cos4/1, Cos2/1
  Cos2/1 -> Product8/2
  [x] -> Product8/1
  Product8/1 -> Add2/1
  [omega] -> Gain9/1
  Gain9/1 -> Cos3/1
  Cos3/1 -> Product9/2
  Cos4/1 -> Product9/1
  Product9/1 -> Add2/2
  Add2/1 -> Divide2/2
  Divide2/1 -> Product10/2
  Product10/1 -> Rt_curise_dot_dot/1  "Rt_curise_dot_dot"
  Derivative/1 -> Derivative1/1
  Derivative1/1 -> Terminator/1  "Rt_curise_der_der"
  Gain8/1 -> Divide2/1

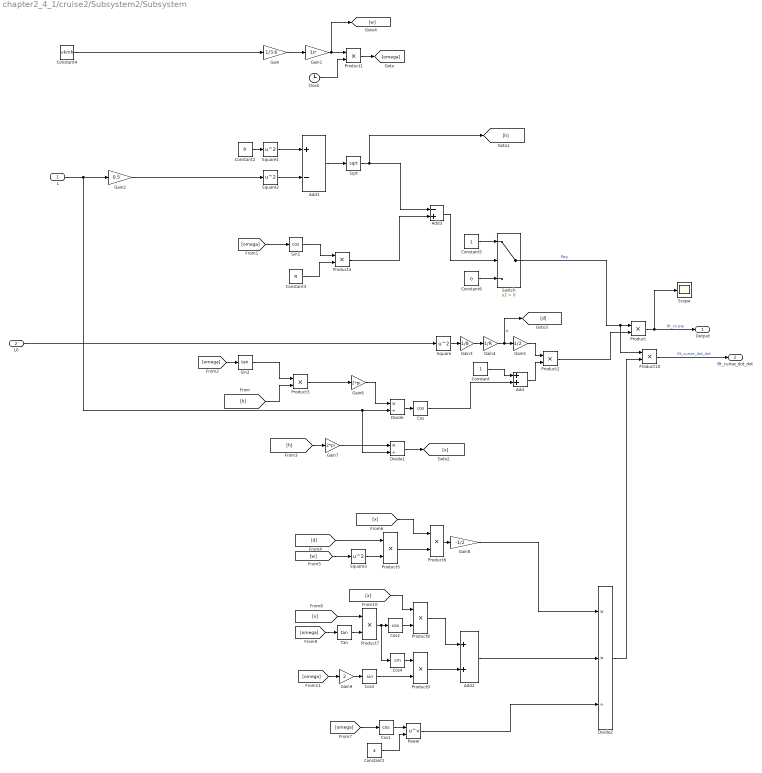
== system chapter2_4_1/cruise2/Subsystem2/Subsystem ==
  L : Inport
  L0 : Inport  Port=2
  Add : Sum
  Add1 : Sum  Inputs=+-
  Add2 : Sum
  Add3 : Sum  Inputs=-+
  Clock : Clock
  Constant : Constant
  Constant1 : Constant  Value=4
  Constant2 : Constant  Value=R
  Constant3 : Constant  Value=R
  Constant4 : Constant  Value=vkmh
  Constant5 : Constant
  Constant6 : Constant  Value=0
  Cos : Trigonometry  Operator=cos
  Cos1 : Trigonometry  Operator=cos
  Cos2 : Trigonometry  Operator=cos
  Cos3 : Trigonometry
  Cos4 : Trigonometry
  Divide : Product  Inputs=*/
  Divide1 : Product  Inputs=*/
  Divide2 : Product  Inputs=**/
  Gain : Gain  Gain=1/3.6
  Gain1 : Gain  Gain=1/r
  Gain2 : Gain  Gain=0.5
  Gain3 : Gain  Gain=1/8
  Gain4 : Gain  Gain=1/R
  Gain5 : Gain  Gain=1/2
  Gain6 : Gain  Gain=2*pi
  Gain7 : Gain  Gain=2*pi
  Gain8 : Gain  Gain=-1/2
  Gain9 : Gain  Gain=2
  Power : Math  Operator=pow
  Product{,1..10} (11 alike) : Product
  Scope : Scope
  Sin1 : Trigonometry  Operator=cos
  Sin2 : Trigonometry  Operator=tan
  Sqrt : Sqrt
  Square{,1..3} (4 alike) : Math  Operator=square
  Switch : Switch  Criteria=u2 > Threshold  SaturateOnIntegerOverflow=off  InputSameDT=off
  Tan : Trigonometry  Operator=tan
  Output : Outport
  Rt_curise_dot_dot : Outport  Port=2
  wires:
  Product10/1 -> Rt_curise_dot_dot/1  "Rt_curise_dot_dot"
  Divide2/1 -> Product10/2
  Add2/1 -> Divide2/2
  Product9/1 -> Add2/2
  Cos4/1 -> Product9/1
  Cos3/1 -> Product9/2
  Gain9/1 -> Cos3/1
  [omega] -> Gain9/1
  Product8/1 -> Add2/1
  [x] -> Product8/1
  Cos2/1 -> Product8/2
  Product7/1 -> Cos2/1, Cos4/1
  [x] -> Product7/1
  Tan/1 -> Product7/2
  [omega] -> Tan/1
  Gain8/1 -> Divide2/1
  Power/1 -> Divide2/3
  Constant1/1 -> Power/2
  Cos1/1 -> Power/1
  [omega] -> Cos1/1
  Product6/1 -> Gain8/1
  [x] -> Product6/1
  Product5/1 -> Product6/2
  [d] -> Product5/1
  Square3/1 -> Product5/2
  [w] -> Square3/1
  Divide1/1 -> [x]
  Gain7/1 -> Divide1/1
  [h] -> Gain7/1
  L/1 -> Gain2/1, Divide/2, Divide1/2
  Constant4/1 -> Gain/1
  Gain6/1 -> Divide/1
  [omega] -> Sin2/1
  Gain2/1 -> Square2/1
  L0/1 -> Square/1
  Constant/1 -> Add/1
  Cos/1 -> Add/2
  Gain5/1 -> Product2/1
  Sin2/1 -> Product3/1
  Product3/1 -> Gain6/1
  Gain1/1 -> Product1/1, [w]
  Product2/1 -> Product/2
  Sqrt/1 -> Add3/1, [h]
  Product/1 -> Scope/1, Output/1  "Rt_crusie"
  Add/1 -> Product2/2
  Sin1/1 -> Product4/1
  Square1/1 -> Add1/1
  Switch/1 -> Product/1, Product10/1  "flag"
  Square2/1 -> Add1/2
  Constant5/1 -> Switch/1
  Gain4/1 -> Gain5/1, [d]  "d"
  Add3/1 -> Switch/2
  Constant3/1 -> Product4/2
  [omega] -> Sin1/1
  [h] -> Product3/2
  Constant6/1 -> Switch/3
  Square/1 -> Gain3/1
  Constant2/1 -> Square1/1
  Product4/1 -> Add3/2
  Gain/1 -> Gain1/1
  Divide/1 -> Cos/1
  Gain3/1 -> Gain4/1
  Add1/1 -> Sqrt/1
  Product1/1 -> [omega]
  Clock/1 -> Product1/2

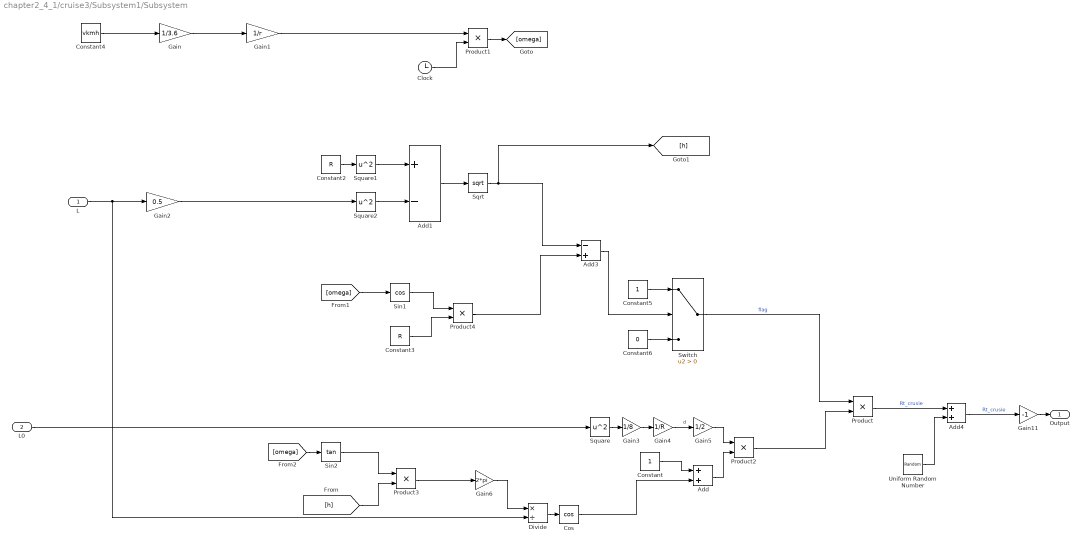
== system chapter2_4_1/cruise3/Subsystem1/Subsystem ==
  L : Inport
  L0 : Inport  Port=2
  Add : Sum
  Add1 : Sum  Inputs=+-
  Add3 : Sum  Inputs=-+
  Add4 : Sum
  Clock : Clock
  Constant : Constant
  Constant2 : Constant  Value=R
  Constant3 : Constant  Value=R
  Constant4 : Constant  Value=vkmh
  Constant5 : Constant
  Constant6 : Constant  Value=0
  Cos : Trigonometry  Operator=cos
  Divide : Product  Inputs=*/
  Gain : Gain  Gain=1/3.6
  Gain1 : Gain  Gain=1/r
  Gain11 : Gain  Gain=-1
  Gain2 : Gain  Gain=0.5
  Gain3 : Gain  Gain=1/8
  Gain4 : Gain  Gain=1/R
  Gain5 : Gain  Gain=1/2
  Gain6 : Gain  Gain=2*pi
  Product{,1..4} (5 alike) : Product
  Sin1 : Trigonometry  Operator=cos
  Sin2 : Trigonometry  Operator=tan
  Sqrt : Sqrt
  Square : Math  Operator=square
  Square1 : Math  Operator=square
  Square2 : Math  Operator=square
  Switch : Switch  Criteria=u2 > Threshold  SaturateOnIntegerOverflow=off  InputSameDT=off
  Uniform Random Number : UniformRandomNumber  Minimum=minRandom  Maximum=maxRandom  SampleTime=1e-3
  Output : Outport
  wires:
  Clock/1 -> Product1/2
  Product1/1 -> [omega]
  Add1/1 -> Sqrt/1
  Gain3/1 -> Gain4/1
  Divide/1 -> Cos/1
  Gain/1 -> Gain1/1
  Product4/1 -> Add3/2
  Constant2/1 -> Square1/1
  Square/1 -> Gain3/1
  Constant6/1 -> Switch/3
  [h] -> Product3/2
  [omega] -> Sin1/1
  Constant3/1 -> Product4/2
  Add3/1 -> Switch/2
  Gain4/1 -> Gain5/1  "d"
  Constant5/1 -> Switch/1
  Square2/1 -> Add1/2
  Switch/1 -> Product/1  "flag"
  Square1/1 -> Add1/1
  Sin1/1 -> Product4/1
  Add/1 -> Product2/2
  Add4/1 -> Gain11/1  "Rt_crusie"
  Sqrt/1 -> [h], Add3/1
  Product2/1 -> Product/2
  Gain1/1 -> Product1/1
  Product3/1 -> Gain6/1
  Sin2/1 -> Product3/1
  Gain5/1 -> Product2/1
  Cos/1 -> Add/2
  Constant/1 -> Add/1
  L0/1 -> Square/1
  Gain2/1 -> Square2/1
  [omega] -> Sin2/1
  Gain6/1 -> Divide/1
  Constant4/1 -> Gain/1
  L/1 -> Divide/2, Gain2/1
  Gain11/1 -> Output/1
  Uniform Random Number/1 -> Add4/2
  Product/1 -> Add4/1  "Rt_crusie"

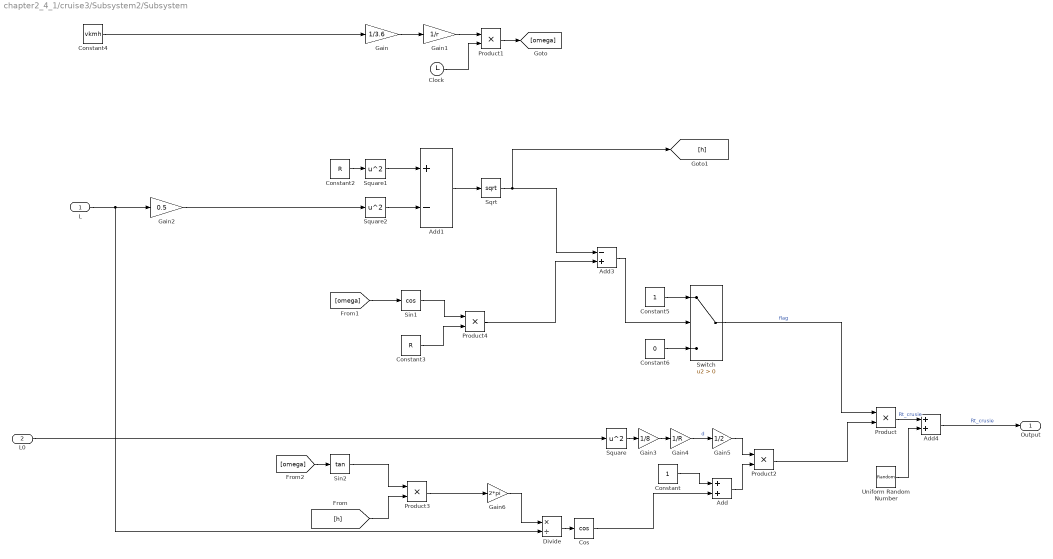
== system chapter2_4_1/cruise3/Subsystem2/Subsystem ==
  L : Inport
  L0 : Inport  Port=2
  Add : Sum
  Add1 : Sum  Inputs=+-
  Add3 : Sum  Inputs=-+
  Add4 : Sum
  Clock : Clock
  Constant : Constant
  Constant2 : Constant  Value=R
  Constant3 : Constant  Value=R
  Constant4 : Constant  Value=vkmh
  Constant5 : Constant
  Constant6 : Constant  Value=0
  Cos : Trigonometry  Operator=cos
  Divide : Product  Inputs=*/
  Gain : Gain  Gain=1/3.6
  Gain1 : Gain  Gain=1/r
  Gain2 : Gain  Gain=0.5
  Gain3 : Gain  Gain=1/8
  Gain4 : Gain  Gain=1/R
  Gain5 : Gain  Gain=1/2
  Gain6 : Gain  Gain=2*pi
  Product{,1..4} (5 alike) : Product
  Sin1 : Trigonometry  Operator=cos
  Sin2 : Trigonometry  Operator=tan
  Sqrt : Sqrt
  Square : Math  Operator=square
  Square1 : Math  Operator=square
  Square2 : Math  Operator=square
  Switch : Switch  Criteria=u2 > Threshold  SaturateOnIntegerOverflow=off  InputSameDT=off
  Uniform Random Number : UniformRandomNumber  Minimum=minRandom  Maximum=maxRandom  Seed=1  SampleTime=1e-3
  Output : Outport
  wires:
  L/1 -> Gain2/1, Divide/2
  Constant4/1 -> Gain/1
  Gain6/1 -> Divide/1
  [omega] -> Sin2/1
  Gain2/1 -> Square2/1
  L0/1 -> Square/1
  Constant/1 -> Add/1
  Cos/1 -> Add/2
  Gain5/1 -> Product2/1
  Sin2/1 -> Product3/1
  Product3/1 -> Gain6/1
  Gain1/1 -> Product1/1
  Product2/1 -> Product/2
  Sqrt/1 -> Add3/1, [h]
  Add4/1 -> Output/1  "Rt_crusie"
  Add/1 -> Product2/2
  Sin1/1 -> Product4/1
  Square1/1 -> Add1/1
  Switch/1 -> Product/1  "flag"
  Square2/1 -> Add1/2
  Constant5/1 -> Switch/1
  Gain4/1 -> Gain5/1  "d"
  Add3/1 -> Switch/2
  Constant3/1 -> Product4/2
  [omega] -> Sin1/1
  [h] -> Product3/2
  Constant6/1 -> Switch/3
  Square/1 -> Gain3/1
  Constant2/1 -> Square1/1
  Product4/1 -> Add3/2
  Gain/1 -> Gain1/1
  Divide/1 -> Cos/1
  Gain3/1 -> Gain4/1
  Add1/1 -> Sqrt/1
  Product1/1 -> [omega]
  Clock/1 -> Product1/2
  Uniform Random Number/1 -> Add4/2
  Product/1 -> Add4/1  "Rt_crusie"
